simulink model "simp_db"  (R2020b)
settings: Solver=VariableStepAuto  StartTime=0.0  StopTime=20  MaxStep=1e-2  RelTol=1e-3
settings Model: Creator=carma  LastModifiedBy=carma

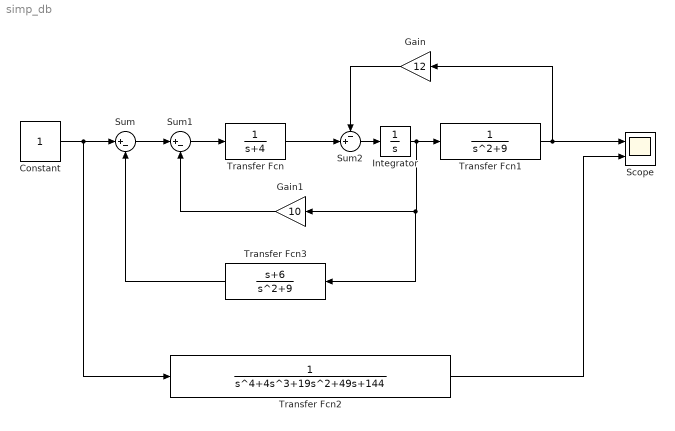
== system simp_db ==
  Constant : Constant  VectorParams1D=off  SampleTime=-1
  Gain : Gain  Gain=12
  Gain1 : Gain  Gain=10
  Integrator : Integrator
  Scope : Scope  NumInputPorts=2
  Sum : Sum  Inputs=|+-
  Sum1 : Sum  Inputs=|+-
  Sum2 : Sum  Inputs=-+|
  Transfer Fcn : TransferFcn  Denominator=[1 4]
  Transfer Fcn1 : TransferFcn  Denominator=[1 0 9]
  Transfer Fcn2 : TransferFcn  Denominator=[1 4 19 49 144]
  Transfer Fcn3 : TransferFcn  Numerator=[1 6]  Denominator=[1 0 9]
  wires:
  Transfer Fcn1/1 -> Gain/1, Scope/1
  Sum/1 -> Sum1/1
  Sum1/1 -> Transfer Fcn/1
  Transfer Fcn/1 -> Sum2/2
  Gain/1 -> Sum2/1
  Sum2/1 -> Integrator/1
  Integrator/1 -> Transfer Fcn3/1, Gain1/1, Transfer Fcn1/1
  Gain1/1 -> Sum1/2
  Transfer Fcn3/1 -> Sum/2
  Constant/1 -> Transfer Fcn2/1, Sum/1
  Transfer Fcn2/1 -> Scope/2
